simulink model "week1prob6"  (R2020b)
settings: Solver=VariableStepAuto  StartTime=0.0  StopTime=10.0  RelTol=1e-3
settings Model: Creator=HP  LastModifiedBy=HP

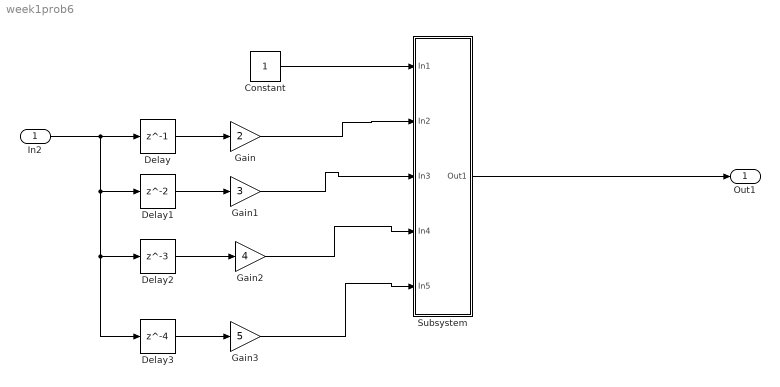
== system week1prob6 ==
  In2 : Inport  OutDataTypeStr=double  PortDimensions=1  SampleTime=[0,1]
  Constant : Constant
  Delay : Delay  DelayLength=1
  Delay1 : Delay
  Delay2 : Delay  DelayLength=3
  Delay3 : Delay  DelayLength=4
  Gain : Gain  Gain=2
  Gain1 : Gain  Gain=3
  Gain2 : Gain  Gain=4
  Gain3 : Gain  Gain=5
  Subsystem : Subsystem
  Out1 : Outport
  wires:
  Subsystem/1(Out1) -> Out1/1
  Delay3/1 -> Gain3/1
  Delay2/1 -> Gain2/1
  Delay1/1 -> Gain1/1
  In2/1 -> Delay3/1, Delay2/1, Delay1/1, Delay/1
  Delay/1 -> Gain/1
  Constant/1 -> Subsystem/1(In1)
  Gain/1 -> Subsystem/2(In2)
  Gain1/1 -> Subsystem/3(In3)
  Gain2/1 -> Subsystem/4(In4)
  Gain3/1 -> Subsystem/5(In5)

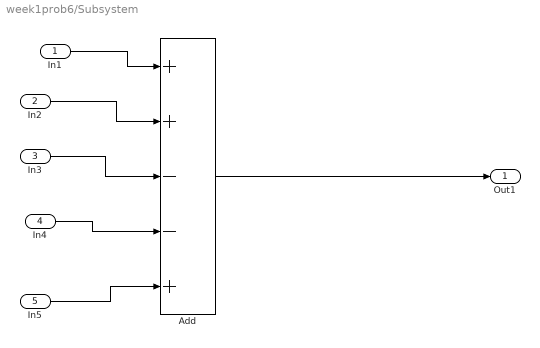
== system week1prob6/Subsystem ==
  In1 : Inport
  In2 : Inport  Port=2
  In3 : Inport  Port=3
  In4 : Inport  Port=4
  In5 : Inport  Port=5
  Add : Sum  Inputs=++--+
  Out1 : Outport
  wires:
  In3/1 -> Add/3
  In2/1 -> Add/2
  In5/1 -> Add/5
  Add/1 -> Out1/1
  In1/1 -> Add/1
  In4/1 -> Add/4
